simulink model "Gen_Sink_RS232_HFC_2P"  (Simulink 7.8)
settings: Solver=VariableStepDiscrete  StartTime=0.0  StopTime=Inf  FixedStep=Ts/4  RelTol=1e-3
PreLoadFcn:
  | clear all;
  | close all;
  | clc;
  | 
  | Ts = 1;          % clk (period)
  | 
  | Ns =  1;      % Characters to Tx and to Rx
StartFcn:
  | clc;
  | close all;
  | 
  | Ns =  100;      % Characters to Tx and to Rx
  | minV = 0;       %  minimum data value
  | maxV = 255;       %  minimum data value
  | Tx_A = randi([minV maxV], 1, Ns, 'uint8');
  | Rx_A = randi([minV maxV], 1, Ns, 'uint8');
  | Tx_B = randi([minV maxV], 1, Ns, 'uint8');
  | Rx_B = randi([minV maxV], 1, Ns, 'uint8');
  | 
  | %
  | %   RS232 ports initialization
  | %
  | PORTNAME1 = 'COM57';
  | fprintf('\nOpening RS232 port %s ...... ', PORTNAME1);
  | s1 = serial(PORTNAME1,'BaudRate',9600,'Parity','none','DataBits',8);
  | set(s1, 'FlowControl', 'none');
  | set(s1, 'InputBufferSize', 64);
  | set(s1, 'OutputBufferSize', 1);
  | fopen(s1);
  | fprintf('\nRS232 port %s activated\n', PORTNAME1);
  | 
  | 
  | PORTNAME2 = 'COM34';
  | fprintf('\nOpening RS232 port %s ...... ', PORTNAME2);
  | s2 = serial(PORTNAME2,'BaudRate',9600,'Parity','none','DataBits',8);
  | set(s2, 'FlowControl', 'none');
  | set(s2, 'InputBufferSize', 64);
  | set(s2, 'OutputBufferSize', 1);
  | fopen(s2);
  | fprintf('\nRS232 port %s activated\n', PORTNAME2);
  | 
  | b2o_s1 = uint8(0);
  | d2o_s1 = uint8(0);
  | b2r_s1 = uint8(0);
  | d2r_s1 = uint8(0);
  | rts_s1 = uint8(0);
  | cts_s1 = uint8(0);
  | 
  | b2o_s2 = uint8(0);
  | d2o_s2 = uint8(0);
  | b2r_s2 = uint8(0);
  | d2r_s2 = uint8(0);
  | rts_s2 = uint8(0);
  | cts_s2 = uint8(0);
StopFcn:
  | %
  | %   RS232 ports release
  | %
  | disp(' ');
  | disp('Deactivating RS232 ports ......');
  | 
  | fclose(s1)
  | delete(s1)
  | clear s1
  | fprintf('RS232 port %s deactivated\n', PORTNAME1);
  | 
  | fclose(s2)
  | delete(s2)
  | clear s2
  | 
  | fprintf('RS232 port %s deactivated\n', PORTNAME2);
  | disp(' ');
  | 
  | if sum(Tx_A == Rx_B) == Ns &&  sum(Tx_B == Rx_A) == Ns
  |   disp('Data exchange without errors');
  | else
  |    NeA = sum((Tx_A - Rx_B) ~= 0);
  |    fprintf('\nA->B:  Data exchange with %d errors in %d data charactes\n\n', NeA, Ns);
  |    NeB = sum((Tx_B - Rx_A) ~= 0);
  |    fprintf('\nB->A:  Data exchange with %d errors in %d data charactes\n\n', NeB, Ns);
  | end
libraries: simulink x5
settings Model: Creator=theodore  LastModifiedBy=theodore
settings DebuggingCC: SolverPrmCheckMsg=none
settings CodeAppCC: CustomSymbolStrType=$N$R$M_T

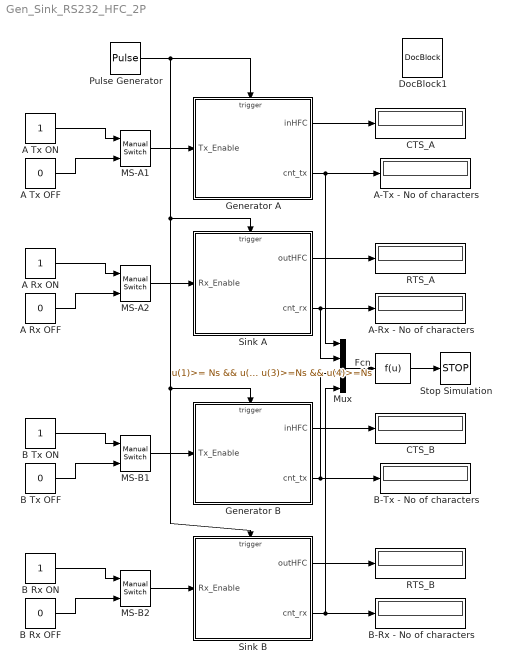
== system Gen_Sink_RS232_HFC_2P ==
  A Rx OFF : Constant  Value=0
  A Rx ON : Constant
  A Tx OFF : Constant  Value=0
  A Tx ON : Constant
  A-Rx - No of characters : Display
  A-Tx - No of characters : Display
  B Rx OFF : Constant  Value=0
  B Rx ON : Constant
  B Tx OFF : Constant  Value=0
  B Tx ON : Constant
  B-Rx - No of characters : Display
  B-Tx - No of characters : Display
  CTS_A : Display
  CTS_B : Display
  DocBlock1 : simulink/Model-Wide Utilities/DocBlock  DocumentType=Text
  Fcn : Fcn  Expr=u(1)>= Ns && u(2)>=Ns && u(3)>=Ns && u(4)>=Ns
  Generator A : Stateflow chart  TreatAsAtomicUnit=on
  Generator B : Stateflow chart  TreatAsAtomicUnit=on
  MS-A1 : simulink/Signal Routing/Manual Switch  sw=1  action=0  varsize=off
  MS-A2 : simulink/Signal Routing/Manual Switch  sw=1  action=0  varsize=off
  MS-B1 : simulink/Signal Routing/Manual Switch  sw=1  action=0  varsize=off
  MS-B2 : simulink/Signal Routing/Manual Switch  sw=1  action=0  varsize=off
  Mux : Mux
  Pulse Generator : DiscretePulseGenerator  PulseType=Time based  Period=Ts  PulseWidth=50
  RTS_A : Display
  RTS_B : Display
  Sink A : Stateflow chart  TreatAsAtomicUnit=on
  Sink B : Stateflow chart  TreatAsAtomicUnit=on
  Stop Simulation : Stop
  wires:
  Pulse Generator/1 -> Generator A/Trigger, Sink A/Trigger, Generator B/Trigger, Sink B/Trigger
  Sink A/2(cnt_rx) -> A-Rx - No of characters/1, Mux/2
  Sink A/1(outHFC) -> RTS_A/1
  Generator A/1(inHFC) -> CTS_A/1
  Generator A/2(cnt_tx) -> A-Tx - No of characters/1, Mux/1
  MS-A1/1 -> Generator A/1(Tx_Enable)
  A Tx ON/1 -> MS-A1/1
  A Tx OFF/1 -> MS-A1/2
  A Rx ON/1 -> MS-A2/1
  A Rx OFF/1 -> MS-A2/2
  MS-A2/1 -> Sink A/1(Rx_Enable)
  Fcn/1 -> Stop Simulation/1
  Mux/1 -> Fcn/1
  Sink B/2(cnt_rx) -> B-Rx - No of characters/1, Mux/4
  Sink B/1(outHFC) -> RTS_B/1
  Generator B/1(inHFC) -> CTS_B/1
  Generator B/2(cnt_tx) -> B-Tx - No of characters/1, Mux/3
  MS-B1/1 -> Generator B/1(Tx_Enable)
  B Tx ON/1 -> MS-B1/1
  B Tx OFF/1 -> MS-B1/2
  B Rx ON/1 -> MS-B2/1
  B Rx OFF/1 -> MS-B2/2
  MS-B2/1 -> Sink B/1(Rx_Enable)

== stateflow chart Sink A ==
  state HFC_states [parallel]
    settings: executionOrder=1
    state HFCcon
      LBstatus_rx = Rx_Enable;
      ml.rts_s1 = LBstatus_rx;
      outHFC = LBstatus_rx;
      ml('RTS_1');
    state S1
      LBstatus_rx = Rx_Enable;
    state S2
    (default) -> HFCcon
    (junction 11) -> S1 [order 1] : [LBstatus_rx == 0]
    S1 -> (junction 12)
    S2 -> HFCcon
    HFCcon -> (junction 11)
    (junction 11) -> HFCcon [order 2]
    (junction 12) -> HFCcon [order 2]
    (junction 12) -> S2 [order 1] : [LBstatus_rx == 0]
  state Rx [parallel]
    settings: executionOrder=2
    state RxState
      en: ml('DIn_1');
      Val_rx = ml.d2r_s1;
      cnt_rx = cnt_rx + 1;
      ml.Rx_A[cnt_rx] = Val_rx;
    state IniState
    (default) -> IniState : {cnt_rx = 0;}
    (junction 10) -> IniState [order 1] : [ml.b2r_s1 == 0 ]
    (junction 10) -> RxState [order 2]
    IniState -> (junction 10) : {ml('B2R_1'); }
    RxState -> IniState
  data: outHFC output double; Val_rx local uint8; cnt_rx output double; LBstatus_rx local double =0; Rx_Enable input double
  events: CLK input RISING_EDGE_EVENT

== stateflow chart Generator B ==
  state Dcalc
    en: ml('CTS_2');
    LBstatus_tx = ml.cts_s2;
    inHFC = LBstatus_tx;
  state IniState
    ml('CTS_2');
    LBstatus_tx = ml.cts_s2;
    inHFC = LBstatus_tx;
  state TxState
    en: cnt_tx = cnt_tx + 1;
    Val_tx = ml.Tx_B[cnt_tx];
    ml.d2o_s2 = Val_tx;
    ml('DOut_2');
  state Idle
  (junction 39) -> TxState [order 1] : [LBstatus_tx  ~= 0  && Tx_Enable == 1 ]
  (junction 38) -> Dcalc [order 2]
  (default) -> IniState : {cnt_tx = 0;}
  (junction 38) -> IniState [order 1] : [ml.b2o_s2 > 0 || LBstatus_tx == 0 || Tx_Enable == 0]
  TxState -> (junction 40)
  IniState -> (junction 38) : {ml('B2O_2'); }
  Dcalc -> (junction 39)
  (junction 39) -> Dcalc [order 2]
  (junction 40) -> Idle [order 1] : [cnt_tx == ml.Ns]
  (junction 40) -> IniState [order 2]
  data: inHFC output double; cnt_tx output double; Val_tx local uint8; LBstatus_tx local double =0; Tx_Enable input double
  events: CLK input RISING_EDGE_EVENT

== stateflow chart Generator A ==
  state Dcalc
    en: ml('CTS_1');
    LBstatus_tx = ml.cts_s1;
    inHFC = LBstatus_tx;
  state IniState
    ml('CTS_1');
    LBstatus_tx = ml.cts_s1;
    inHFC = LBstatus_tx;
  state TxState
    en: cnt_tx = cnt_tx + 1;
    Val_tx = ml.Tx_A[cnt_tx];
    ml.d2o_s1 = Val_tx;
    ml('DOut_1');
  state Idle
  (junction 64) -> TxState [order 1] : [LBstatus_tx  ~= 0  && Tx_Enable == 1 ]
  (junction 63) -> Dcalc [order 2]
  (default) -> IniState : {cnt_tx = 0;}
  (junction 63) -> IniState [order 1] : [ml.b2o_s1 > 0 || LBstatus_tx == 0 || Tx_Enable == 0]
  TxState -> (junction 65)
  IniState -> (junction 63) : {ml('B2O_1'); }
  Dcalc -> (junction 64)
  (junction 64) -> Dcalc [order 2]
  (junction 65) -> Idle [order 1] : [cnt_tx == ml.Ns]
  (junction 65) -> IniState [order 2]
  data: inHFC output double; cnt_tx output double; Val_tx local uint8; LBstatus_tx local double =0; Tx_Enable input double
  events: CLK input RISING_EDGE_EVENT

== stateflow chart Sink B ==
  state HFC_states [parallel]
    settings: executionOrder=1
    state HFCcon
      LBstatus_rx = Rx_Enable;
      ml.rts_s2 = LBstatus_rx;
      outHFC = LBstatus_rx;
      ml('RTS_2');
    state S1
      LBstatus_rx = Rx_Enable;
    state S2
    (default) -> HFCcon
    (junction 92) -> S1 [order 1] : [LBstatus_rx == 0]
    S1 -> (junction 93)
    S2 -> HFCcon
    HFCcon -> (junction 92)
    (junction 92) -> HFCcon [order 2]
    (junction 93) -> HFCcon [order 2]
    (junction 93) -> S2 [order 1] : [LBstatus_rx == 0]
  state Rx [parallel]
    settings: executionOrder=2
    state RxState
      en: ml('DIn_2');
      Val_rx = ml.d2r_s2;
      cnt_rx = cnt_rx + 1;
      ml.Rx_B[cnt_rx] = Val_rx;
    state IniState
    (default) -> IniState : {cnt_rx = 0;}
    (junction 91) -> IniState [order 1] : [ml.b2r_s2 == 0 ]
    (junction 91) -> RxState [order 2]
    IniState -> (junction 91) : {ml('B2R_2'); }
    RxState -> IniState
  data: outHFC output double; Val_rx local uint8; cnt_rx output double; LBstatus_rx local double =0; Rx_Enable input double
  events: CLK input RISING_EDGE_EVENT
